simulink model "lab_6_task_2_simulink"  (R2025b)
settings: Solver=ode4  StartTime=0.0  StopTime=10  FixedStep=0.001  RelTol=1e-3
values from neighbouring files (symbols this model uses):
  ABN0 = eye(3)    [lab_6_task_1.m]    (also in lab_6_task_2.m)
  I = diag([ix iy iz])    [lab_4_task_1.m]    (also in lab_5_task_1.m; lab_5_task_2.m; lab_6_task_1.m = diag([ ix iy iz ]); lab_6_task_2.m = diag([ ix iy iz ]))
  mu_E = astroConstants(13)    [lab_6_task_2.m]    (also in lab_7_task_1.m; lab_7_task_2.m)
  n = sqrt(G*M_e/R^3)    [lab_6_task_1.m]    (also in lab_6_task_2.m; lab_7_task_1.m = sqrt(mu_E/(a^3)); lab_7_task_2.m = sqrt(mu_E/(a^3)); lab_7_task_3.m = sqrt(mu/(a^3)))
  R = A(:,:,i)    [animate_frame.m]    (also in lab_6_task_1.m = 6771; lab_6_task_2.m = 6771)
  w0 = [0.01 0.01 0.01]    [lab_3_task_3.m]    (also in lab_5_task_1.m = [wx0 wy0 wz0]; lab_5_task_2.m = [wx0 wy0 wz0]; lab_6_task_1.m = [wx0 wy0 wz0]; lab_6_task_2.m = [wx0 wy0 wz0])
  wLN = [0; 0; n;]    [lab_6_task_2.m]
libraries: matrix_library x2
settings Model: Creator=nicol  LastModifiedBy=User

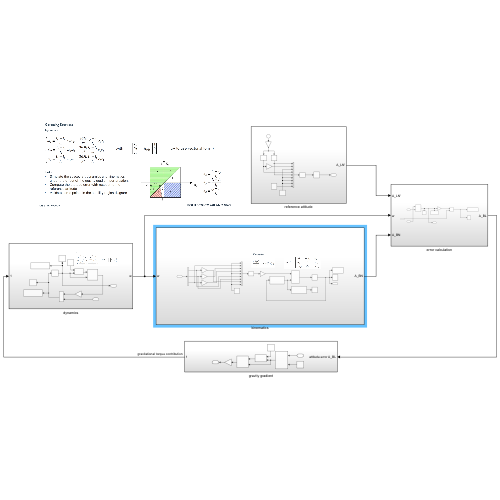
[thumbnail: Simulink's stored preview of the top-level diagram]
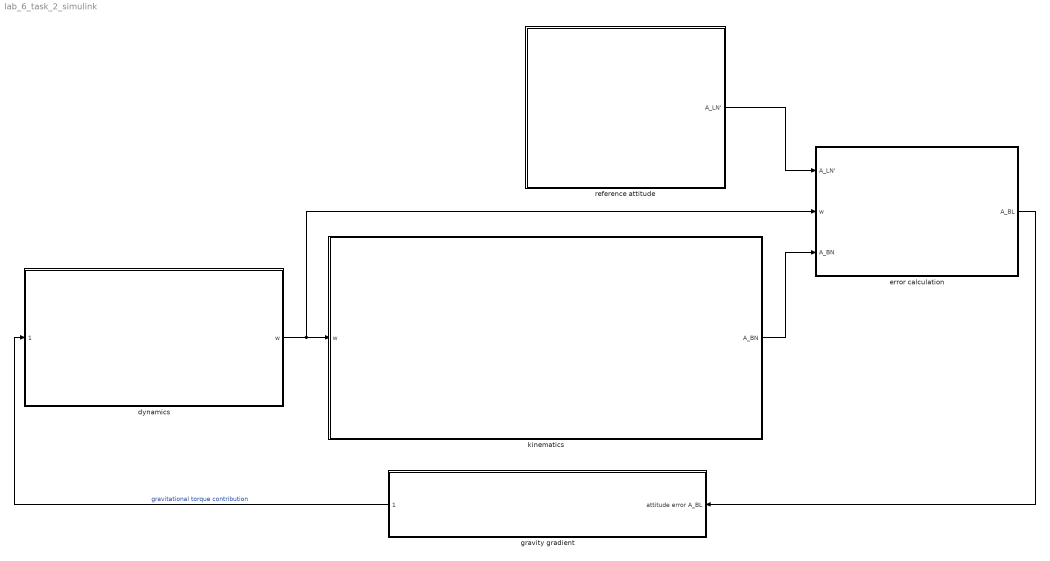
== system lab_6_task_2_simulink ==
  dynamics : Subsystem
  error calculation : Subsystem
  gravity gradient : Subsystem
      settings: PortSchema="{\"entries\":[{\"content\":{\"sides\":[{\"content\":{\"connectorIds\":[\"Out1\"]},\"type\":\"ConnectorPlacement.EquallySpacedRectSide\",\"uuid\":\"2a67419a-68c9-4369-a698-e6ac26417455\"},{\"content\":{\"connectorIds\":[\"In1\"],\"side\":\"RIGHT\"},\"type\":\"ConnectorPlacement.EquallySpacedRectSide\",\"uuid\":\"5f3f4c4a-6b79-4b92-8f4c-19ffa36753b2\"},{\"content\":{\"side\":\"TOP\"},\"type\":\"ConnectorPlacement.EquallySpacedRectSide\",\"uuid\":\"22c946b7-ea77-4444-a63c-d5b3d585f671\"}]},\"type\":\"ConnectorPlacement.EquallySpacedConnector\",\"uuid\":\"037c4a72-b28b-418e-a921-9da68dc0cd93\"}],\"packageUris\":[\"http://schema.mathworks.com/mf0/Connector/R2020b\"],\"version\":\"1.0\"}"
  kinematics : Subsystem
  reference attitude : Subsystem
  wires:
  dynamics/1(w) -> error calculation/2(w), kinematics/1(w)
  reference attitude/1(A_LN') -> error calculation/1(A_LN')
  kinematics/1(A_BN) -> error calculation/3(A_BN)
  error calculation/1(A_BL) -> gravity gradient/1(attitude error A_BL)
  gravity gradient/1(1) -> dynamics/1(1)  "gravitational torque contribution"

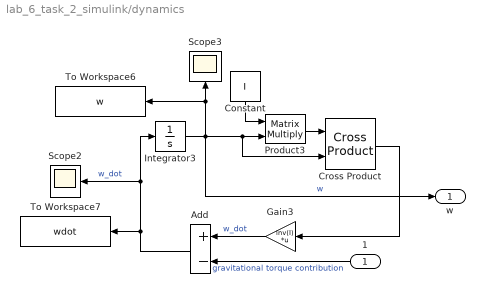
== system lab_6_task_2_simulink/dynamics ==
  1 : Inport
  Add : Sum  Inputs=+-
  Constant : Constant  Value=I
  Cross Product : matrix_library/Cross Product
  Gain3 : Gain  Gain=inv(I)  Multiplication=Matrix(K*u)
  Integrator3 : Integrator  InitialCondition=w0
  Product3 : Product  Multiplication=Matrix(*)
  Scope2 : Scope
      settings: ActiveDisplayYMinimum=-1  ActiveDisplayYMaximum=1  DataLoggingVariableName=ScopeData2
  Scope3 : Scope
      settings: ActiveDisplayYMinimum=-1  ActiveDisplayYMaximum=1  DataLoggingVariableName=ScopeData3
  To Workspace6 : ToWorkspace  VariableName=w  SaveFormat=Timeseries  SampleTime=-1
  To Workspace7 : ToWorkspace  VariableName=wdot  SaveFormat=Timeseries  SampleTime=-1
  w : Outport
  wires:
  Integrator3/1 -> w/1, Cross Product/2, Product3/2, To Workspace6/1, Scope3/1  "w"
  Cross Product/1 -> Gain3/1
  Add/1 -> Scope2/1, Integrator3/1, To Workspace7/1  "w_dot"
  Product3/1 -> Cross Product/1
  Constant/1 -> Product3/1
  Gain3/1 -> Add/1  "w_dot"
  1/1 -> Add/2  "gravitational torque contribution"

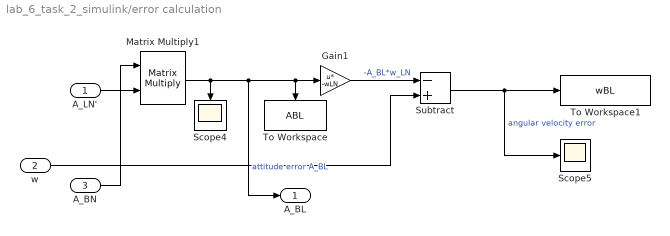
== system lab_6_task_2_simulink/error calculation ==
  A_LN' : Inport
  w : Inport  Port=2
  A_BN : Inport  Port=3
  Gain1 : Gain  Gain=-wLN  Multiplication=Matrix(u*K)
  Matrix Multiply1 : Product  Multiplication=Matrix(*)
  Scope4 : Scope
      settings: ActiveDisplayYMinimum=-0.80513740299452052  ActiveDisplayYMaximum=1.2005708225549467  DataLoggingVariableName=ScopeData4
  Scope5 : Scope
      settings: ActiveDisplayYMinimum=-8.953871770327698  ActiveDisplayYMaximum=80.584845932949293  DataLoggingVariableName=ScopeData5
  Subtract : Sum  Inputs=-+
  To Workspace : ToWorkspace  VariableName=ABL  SaveFormat=Timeseries  SampleTime=-1
  To Workspace1 : ToWorkspace  VariableName=wBL  SaveFormat=Timeseries  SampleTime=-1
  A_BL : Outport
  wires:
  Subtract/1 -> Scope5/1, To Workspace1/1  "angular velocity error"
  A_BN/1 -> Matrix Multiply1/1
  Matrix Multiply1/1 -> A_BL/1, To Workspace/1, Gain1/1, Scope4/1  "attitude error A_BL"
  A_LN'/1 -> Matrix Multiply1/2
  Gain1/1 -> Subtract/1  "-A_BL*w_LN"
  w/1 -> Subtract/2

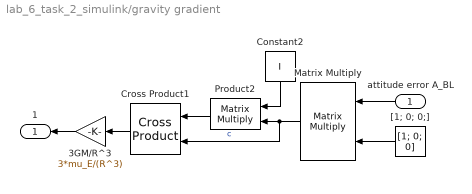
== system lab_6_task_2_simulink/gravity gradient ==
  attitude error A_BL : Inport
  3GM/R^3 : Gain  Gain=3*mu_E/(R^3)
  Constant2 : Constant  Value=I
  Cross Product1 : matrix_library/Cross Product
  Matrix Multiply : Product  Multiplication=Matrix(*)
  Product2 : Product  Multiplication=Matrix(*)
  "[1; 0; 0;]" : Constant  Value=[1; 0; 0]
  1 : Outport
  wires:
  Matrix Multiply/1 -> Cross Product1/2, Product2/2  "c"
  attitude error A_BL/1 -> Matrix Multiply/1
  Constant2/1 -> Product2/1
  Cross Product1/1 -> 3GM/R^3/1
  Product2/1 -> Cross Product1/1
  "[1; 0; 0;]"/1 -> Matrix Multiply/2
  3GM/R^3/1 -> 1/1

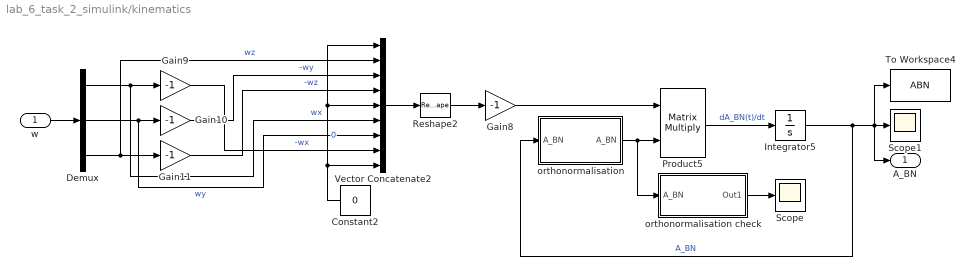
== system lab_6_task_2_simulink/kinematics ==
  w : Inport
  Constant2 : Constant  Value=0
  Demux : Demux  Outputs=3
  Gain{8..11} (4 alike) : Gain  Gain=-1
  Integrator5 : Integrator  InitialCondition=ABN0
  Product5 : Product  Multiplication=Matrix(*)
  Reshape2 : Reshape  OutputDimensionality=Customize  OutputDimensions=[3,3]
  Scope : Scope
      settings: ActiveDisplayYMinimum=-1  ActiveDisplayYMaximum=1
  Scope1 : Scope
      settings: ActiveDisplayYMinimum=-0.12499999999999997  ActiveDisplayYMaximum=1.125
  To Workspace4 : ToWorkspace  VariableName=ABN  SaveFormat=Timeseries  SampleTime=-1
  Vector Concatenate2 : Concatenate  NumInputs=9
  orthonormalisation : Subsystem
  orthonormalisation check : Subsystem
  A_BN : Outport
  wires:
  Product5/1 -> Integrator5/1  "dA_BN(t)/dt"
  Gain11/1 -> Vector Concatenate2/4  "-wz"
  Integrator5/1 -> A_BN/1, To Workspace4/1, Scope1/1, orthonormalisation/1(A_BN)  "A_BN"
  Gain8/1 -> Product5/1
  Demux/1 -> Vector Concatenate2/6, Gain9/1  "wx"
  Reshape2/1 -> Gain8/1
  Gain10/1 -> Vector Concatenate2/3  "-wy"
  Demux/2 -> Vector Concatenate2/7, Gain10/1  "wy"
  Vector Concatenate2/1 -> Reshape2/1
  Demux/3 -> Vector Concatenate2/2, Gain11/1  "wz"
  Constant2/1 -> Vector Concatenate2/1, Vector Concatenate2/5, Vector Concatenate2/9  "0"
  Gain9/1 -> Vector Concatenate2/8  "-wx"
  w/1 -> Demux/1
  orthonormalisation/1(" A_BN") -> Product5/2, orthonormalisation check/1(A_BN)
  orthonormalisation check/1(Out1) -> Scope/1

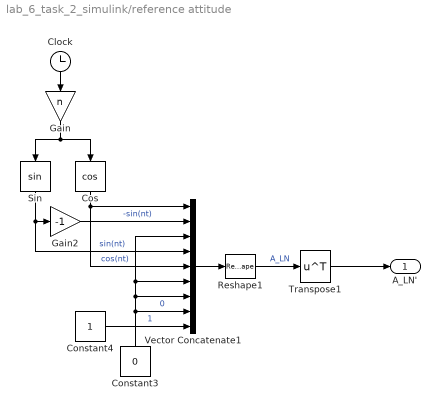
== system lab_6_task_2_simulink/reference attitude ==
  Clock : Clock
  Constant3 : Constant  Value=0
  Constant4 : Constant
  Cos : Trigonometry  Operator=cos
  Gain : Gain  Gain=n
  Gain2 : Gain  Gain=-1
  Reshape1 : Reshape  OutputDimensionality=Customize  OutputDimensions=[3,3]
  Sin : Trigonometry
  Transpose1 : Math  Operator=transpose
  Vector Concatenate1 : Concatenate  NumInputs=9
  A_LN' : Outport
  wires:
  Constant3/1 -> Vector Concatenate1/8, Vector Concatenate1/7, Vector Concatenate1/6, Vector Concatenate1/3  "0"
  Gain/1 -> Sin/1, Cos/1
  Gain2/1 -> Vector Concatenate1/2  "-sin(nt)"
  Sin/1 -> Vector Concatenate1/4, Gain2/1  "sin(nt)"
  Reshape1/1 -> Transpose1/1  "A_LN"
  Clock/1 -> Gain/1
  Cos/1 -> Vector Concatenate1/5, Vector Concatenate1/1  "cos(nt)"
  Vector Concatenate1/1 -> Reshape1/1
  Constant4/1 -> Vector Concatenate1/9  "1"
  Transpose1/1 -> A_LN'/1

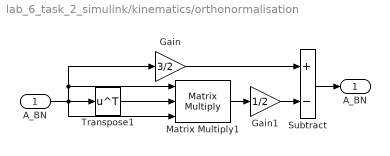
== system lab_6_task_2_simulink/kinematics/orthonormalisation ==
  A_BN : Inport
  Gain : Gain  Gain=3/2
  Gain1 : Gain  Gain=1/2
  Matrix Multiply1 : Product  Inputs=3  Multiplication=Matrix(*)
  Subtract : Sum  Inputs=+-
  Transpose1 : Math  Operator=transpose
  " A_BN" : Outport
  wires:
  Gain/1 -> Subtract/1
  Transpose1/1 -> Matrix Multiply1/2
  Matrix Multiply1/1 -> Gain1/1
  Gain1/1 -> Subtract/2
  Subtract/1 -> " A_BN"/1
  A_BN/1 -> Matrix Multiply1/1, Gain/1, Transpose1/1, Matrix Multiply1/3

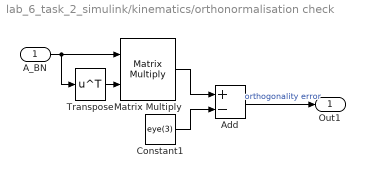
== system lab_6_task_2_simulink/kinematics/orthonormalisation check ==
  A_BN : Inport
  Add : Sum  Inputs=+-
  Constant1 : Constant  Value=eye(3)
  Matrix Multiply : Product  Multiplication=Matrix(*)
  Transpose : Math  Operator=transpose
  Out1 : Outport
  wires:
  Transpose/1 -> Matrix Multiply/2
  A_BN/1 -> Matrix Multiply/1, Transpose/1
  Add/1 -> Out1/1  "orthogonality error"
  Constant1/1 -> Add/2
  Matrix Multiply/1 -> Add/1
